simulink model "FaultCheck"  (R2022b)
settings: Solver=FixedStepAuto  StartTime=0.0  StopTime=10  FixedStep=1  RelTol=1e-3
undefined symbols (not defined in the file): C_Flt_IGBTULowerTempConfirmTh_u16, C_Flt_IGBTULowerTempDiagEn_b, C_Flt_IGBTULowerTempErrCode_u16, C_Flt_IGBTULowerTempPowerCoeff, C_Flt_IGBTULowerTempRecoveryTh_u16, C_Flt_IGBTULowerTempRecTh_s32, C_Flt_IGBTULowerTempTrigTh_s32, C_Flt_IGBTUOverTempConfirmTh_u16, C_Flt_IGBTUOverTempDiagEn_b, C_Flt_IGBTUOverTempErrCode_u16, C_Flt_IGBTUOverTempRecoveryTh_u16, C_Flt_IGBTUOverTempRecTh_s32, C_Flt_IGBTUOverTempTrigTh_s32, C_Flt_IGBTVLowerTempConfirmTh_u16, C_Flt_IGBTVLowerTempDiagEn_b, C_Flt_IGBTVLowerTempErrCode_u16, C_Flt_IGBTVLowerTempPowerCoeff, C_Flt_IGBTVLowerTempRecoveryTh_u16, C_Flt_IGBTVLowerTempRecTh_s32, C_Flt_IGBTVLowerTempTrigTh_s32, C_Flt_IGBTVOverTempConfirmTh_u16, C_Flt_IGBTVOverTempDiagEn_b, C_Flt_IGBTVOverTempErrCode_u16, C_Flt_IGBTVOverTempRecoveryTh_u16, C_Flt_IGBTVOverTempRecTh_s32, C_Flt_IGBTVOverTempTrigTh_s32, C_Flt_IGBTWLowerTempConfirmTh_u16, C_Flt_IGBTWLowerTempDiagEn_b, C_Flt_IGBTWLowerTempErrCode_u16, C_Flt_IGBTWLowerTempPowerCoeff, C_Flt_IGBTWLowerTempRecoveryTh_u16, C_Flt_IGBTWLowerTempRecTh_s32, C_Flt_IGBTWLowerTempTrigTh_s32, C_Flt_IGBTWOverTempConfirmTh_u16, C_Flt_IGBTWOverTempDiagEn_b, C_Flt_IGBTWOverTempErrCode_u16, C_Flt_IGBTWOverTempRecoveryTh_u16, C_Flt_IGBTWOverTempRecTh_s32, C_Flt_IGBTWOverTempTrigTh_s32, C_Flt_IuOCConfirmTh_u16, C_Flt_IuOCDiagEn_b, C_Flt_IuOCErrCode_u16, C_Flt_IuOCNegLimit_s32, C_Flt_IuOCPosLimit_s32, C_Flt_IuOCRecoveryTh_u16, C_Flt_IuZeroDriftDiagEn_b, C_Flt_IuZeroDriftErrCode_u16, C_Flt_IvOCConfirmTh_u16, C_Flt_IvOCDiagEn_b, C_Flt_IvOCErrCode_u16, C_Flt_IvOCNegLimit_s32, C_Flt_IvOCPosLimit_s32, C_Flt_IvOCRecoveryTh_u16, C_Flt_IvZeroDriftDiagEn_b, C_Flt_IvZeroDriftErrCode_u16, C_Flt_IwOCConfirmTh_u16, C_Flt_IwOCDiagEn_b, C_Flt_IwOCErrCode_u16, C_Flt_IwOCNegLimit_s32, C_Flt_IwOCPosLimit_s32 ... (+196)
libraries: YS_UserDefined_Library x21, simulink x5
(part 4 of 11)

== system FaultCheck/FaultDiag_HighTask_100us/FltDetn/UdcDetn/Parameter2 ==
  IPC_UdcRaw_V : Inport
  Bus Creator : BusCreator  Inputs=8
  Constant11 : Constant  Value=Flt_UdcOverLim1_ErrCode
  Constant13 : Constant  Value=FLTLVL_TWO
  Constant2 : Constant  Value=Flt_UdcOverLim1_RecLim1
  Constant3 : Constant  Value=Flt_UdcOverLim1_RecDeb
  Constant6 : Constant  Value=Flt_UdcOverLim1_ActvErrDetn
  Constant7 : Constant  Value=Flt_UdcOverLim1_OverLim1
  Constant8 : Constant  Value=Flt_UdcOverLim1_ErrDeb
  Flt_UdcOverLim1_PowRecCoef : Lookup_n-D  NumberOfTableDimensions=1  BreakpointsForDimension1=Flt_UdcRawOver1_V  BreakpointsForDimension1DataTypeStr=Inherit: Inherit from 'Breakpoint data'  Table=Flt_UdcOverLim1_PowRecCoef  TableDataTypeStr=Inherit: Inherit from 'Table data'  ExtrapMethod=Clip  UseLastTableValue=on  InternalRulePriority=Speed  OutDataTypeStr=single  RndMeth=Simplest
  Para : Outport
  wires:
  IPC_UdcRaw_V/1 -> Flt_UdcOverLim1_PowRecCoef/1
  Bus Creator/1 -> Para/1
  Constant11/1 -> Bus Creator/6  "ErrCode"
  Constant13/1 -> Bus Creator/7  "FltLvl"
  Flt_UdcOverLim1_PowRecCoef/1 -> Bus Creator/8  "PowRecCoef"
  Constant7/1 -> Bus Creator/1  "OverLim1"
  Constant8/1 -> Bus Creator/2  "ErrDeb"
  Constant6/1 -> Bus Creator/3  "ActvnDetn"
  Constant3/1 -> Bus Creator/5  "RecDeb"
  Constant2/1 -> Bus Creator/4  "RecLim1"

== system FaultCheck/FaultDiag_HighTask_100us/FltDetn/UdcDetn/Parameter3 ==
  Bus Creator : BusCreator  Inputs=6
  Constant1 : Constant  Value=FLT_COEF_ZERO
  Constant11 : Constant  Value=Flt_UdcOverLim2_ErrCode
  Constant13 : Constant  Value=FLTLVL_FIVE
  Constant6 : Constant  Value=Flt_UdcOverLim2_ActvErrDetn
  Constant7 : Constant  Value=Flt_UdcOverLim2_OverLim2
  Constant8 : Constant  Value=Flt_UdcOverLim2_ErrDeb
  Para : Outport
  wires:
  Bus Creator/1 -> Para/1
  Constant11/1 -> Bus Creator/4  "ErrCode"
  Constant13/1 -> Bus Creator/5  "FltLvl"
  Constant1/1 -> Bus Creator/6  "PowRecCoef"
  Constant7/1 -> Bus Creator/1  "OverLim2"
  Constant8/1 -> Bus Creator/2  "ErrDeb"
  Constant6/1 -> Bus Creator/3  "ActvnDetn"

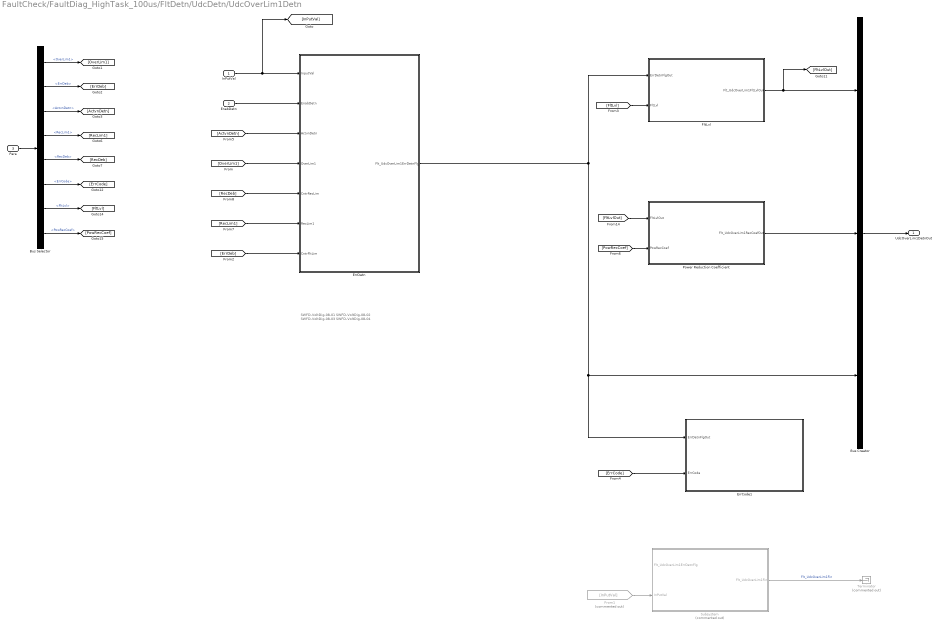
== system FaultCheck/FaultDiag_HighTask_100us/FltDetn/UdcDetn/UdcOverLim1Detn ==
  note: SWFD-VoltDig-08-01
      |
      | SWFD-VoltDig-08-02
      |
      | SWFD-VoltDig-08-03
      |
      | SWFD-VoltDig-08-04
  InPutVal : Inport
  EnabDetn : Inport  Port=2
  Para : Inport  Port=3
  Bus Creator : BusCreator  Inputs=3
  Bus Selector : BusSelector  OutputSignals=OverLim1,ErrDeb,ActvnDetn,RecLim1,RecDeb,ErrCode,FltLvl,PowRecCoef
  ErrCode1 : Subsystem
  ErrDetn : Subsystem
  FltLvl : Subsystem
  From1 : From  Commented=on  GotoTag=InPutVal
  Power Reduction Coefficient : Subsystem
  Subsystem : Subsystem  Commented=on
  Terminator : Terminator  Commented=on
  UdcOverLim1DetnOut : Outport
  wires:
  ErrDetn/1(Flt_UdcOverLim1ErrDetnFlg) -> FltLvl/1(ErrDetnFlgOut), Bus Creator/3, ErrCode1/1(ErrDetnFlgOut)
  Subsystem/1(Flt_UdcOverLim1Fin) -> Terminator/1  "Flt_UdcOverLim1Fin"
  From1/1 -> Subsystem/2(InPutVal)
  Bus Selector/1 -> [OverLim1]  "<OverLim1>"
  Para/1 -> Bus Selector/1
  Bus Selector/3 -> [ActvnDetn]  "<ActvnDetn>"
  Bus Selector/2 -> [ErrDeb]  "<ErrDeb>"
  Bus Selector/4 -> [RecLim1]  "<RecLim1>"
  Bus Selector/5 -> [RecDeb]  "<RecDeb>"
  FltLvl/1(Flt_UdcOverLim1FltLvlOut) -> Bus Creator/1, [FltLvlOut]
  Bus Selector/6 -> [ErrCode]  "<ErrCode>"
  Bus Selector/7 -> [FltLvl]  "<FltLvl>"
  Bus Selector/8 -> [PowRecCoef]  "<PowRecCoef>"
  [FltLvl] -> FltLvl/2(FltLvl)
  [PowRecCoef] -> Power Reduction Coefficient/2(PowRecCoef)
  [FltLvlOut] -> Power Reduction Coefficient/1(FltLvlOut)
  InPutVal/1 -> ErrDetn/1(InputVal), [InPutVal]
  [OverLim1] -> ErrDetn/4(OverLim1)
  EnabDetn/1 -> ErrDetn/2(EnabDetn)
  [ActvnDetn] -> ErrDetn/3(ActvnDetn)
  Power Reduction Coefficient/1(Flt_UdcOverLim1RecCoefOut) -> Bus Creator/2
  Bus Creator/1 -> UdcOverLim1DetnOut/1
  [RecDeb] -> ErrDetn/5(CntrRecLim)
  [RecLim1] -> ErrDetn/6(RecLim1)
  [ErrDeb] -> ErrDetn/7(CntrFltLim)
  [ErrCode] -> ErrCode1/2(ErrCode)

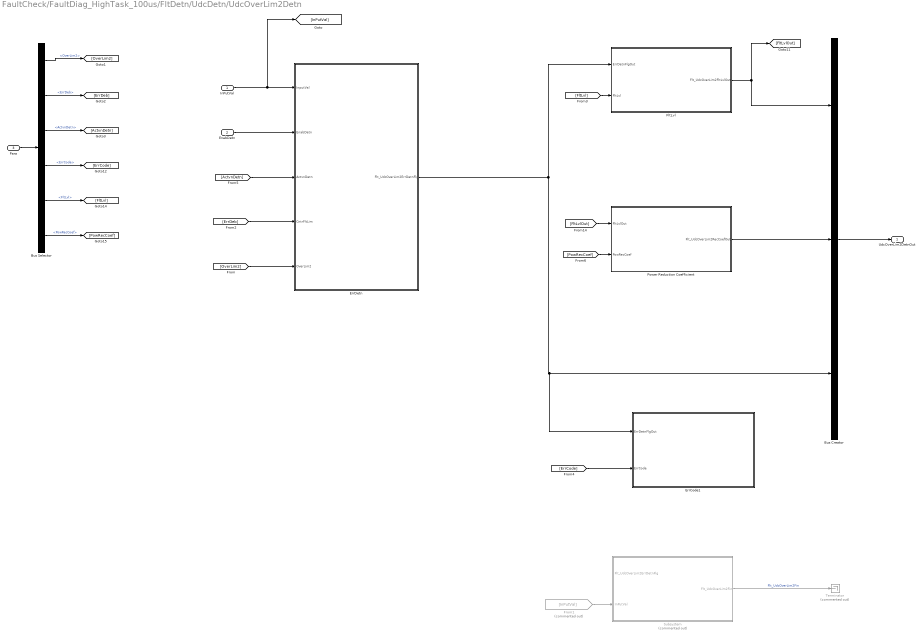
== system FaultCheck/FaultDiag_HighTask_100us/FltDetn/UdcDetn/UdcOverLim2Detn ==
  InPutVal : Inport
  EnabDetn : Inport  Port=2
  Para : Inport  Port=3
  Bus Creator : BusCreator  Inputs=3
  Bus Selector : BusSelector  OutputSignals=OverLim2,ErrDeb,ActvnDetn,ErrCode,FltLvl,PowRecCoef
  ErrCode1 : Subsystem
  ErrDetn : Subsystem
  FltLvl : Subsystem
  From1 : From  Commented=on  GotoTag=InPutVal
  Power Reduction Coefficient : Subsystem
  Subsystem : Subsystem  Commented=on
  Terminator : Terminator  Commented=on
  UdcOverLim2DetnOut : Outport
  wires:
  ErrDetn/1(Flt_UdcOverLim2ErrDetnFlg) -> ErrCode1/1(ErrDetnFlgOut), Bus Creator/3, FltLvl/1(ErrDetnFlgOut)
  From1/1 -> Subsystem/2(InPutVal)
  Subsystem/1(Flt_UdcOverLim2Fin) -> Terminator/1  "Flt_UdcOverLim2Fin"
  [ErrDeb] -> ErrDetn/4(CntrFltLim)
  Bus Creator/1 -> UdcOverLim2DetnOut/1
  Power Reduction Coefficient/1(Flt_UdcOverLim2RecCoefOut) -> Bus Creator/2
  [ActvnDetn] -> ErrDetn/3(ActvnDetn)
  EnabDetn/1 -> ErrDetn/2(EnabDetn)
  [OverLim2] -> ErrDetn/5(OverLim2)
  InPutVal/1 -> ErrDetn/1(InputVal), [InPutVal]
  [FltLvlOut] -> Power Reduction Coefficient/1(FltLvlOut)
  [PowRecCoef] -> Power Reduction Coefficient/2(PowRecCoef)
  [FltLvl] -> FltLvl/2(FltLvl)
  Bus Selector/6 -> [PowRecCoef]  "<PowRecCoef>"
  Bus Selector/5 -> [FltLvl]  "<FltLvl>"
  Bus Selector/4 -> [ErrCode]  "<ErrCode>"
  FltLvl/1(Flt_UdcOverLim2FltLvlOut) -> [FltLvlOut], Bus Creator/1
  Bus Selector/2 -> [ErrDeb]  "<ErrDeb>"
  Bus Selector/3 -> [ActvnDetn]  "<ActvnDetn>"
  Bus Selector/1 -> [OverLim2]  "<OverLim2>"
  Para/1 -> Bus Selector/1
  [ErrCode] -> ErrCode1/2(ErrCode)

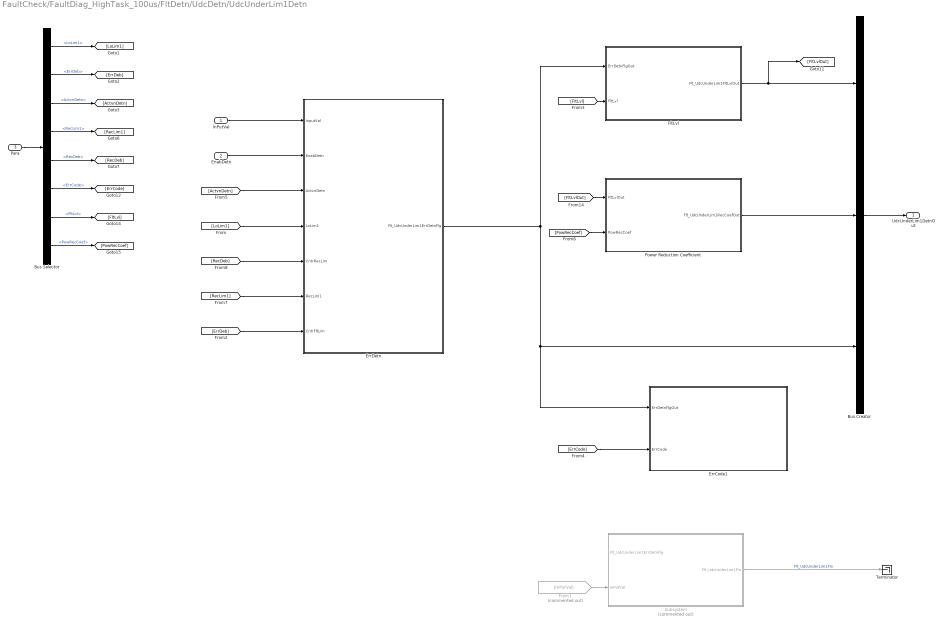
== system FaultCheck/FaultDiag_HighTask_100us/FltDetn/UdcDetn/UdcUnderLim1Detn ==
  InPutVal : Inport
  EnabDetn : Inport  Port=2
  Para : Inport  Port=3
  Bus Creator : BusCreator  Inputs=3
  Bus Selector : BusSelector  OutputSignals=LoLim1,ErrDeb,ActvnDetn,RecLim1,RecDeb,ErrCode,FltLvl,PowRecCoef
  ErrCode1 : Subsystem
  ErrDetn : Subsystem
  FltLvl : Subsystem
  From1 : From  Commented=on  GotoTag=InPutVal
  Power Reduction Coefficient : Subsystem
  Subsystem : Subsystem  Commented=on
  Terminator : Terminator
  UdcUnderLim1DetnOut : Outport
  wires:
  Subsystem/1(Flt_UdcUnderLim1Fin) -> Terminator/1  "Flt_UdcUnderLim1Fin"
  From1/1 -> Subsystem/2(InPutVal)
  ErrDetn/1(Flt_UdcUnderLim1ErrDetnFlg) -> Bus Creator/3, ErrCode1/1(ErrDetnFlgOut), FltLvl/1(ErrDetnFlgOut)
  [ErrDeb] -> ErrDetn/7(CntrFltLim)
  [RecLim1] -> ErrDetn/6(RecLim1)
  [RecDeb] -> ErrDetn/5(CntrRecLim)
  Bus Creator/1 -> UdcUnderLim1DetnOut/1
  Power Reduction Coefficient/1(Flt_UdcUnderLim1RecCoefOut) -> Bus Creator/2
  [ActvnDetn] -> ErrDetn/3(ActvnDetn)
  EnabDetn/1 -> ErrDetn/2(EnabDetn)
  [LoLim1] -> ErrDetn/4(LoLim1)
  InPutVal/1 -> ErrDetn/1(InputVal)
  [FltLvlOut] -> Power Reduction Coefficient/1(FltLvlOut)
  [PowRecCoef] -> Power Reduction Coefficient/2(PowRecCoef)
  [FltLvl] -> FltLvl/2(FltLvl)
  Bus Selector/8 -> [PowRecCoef]  "<PowRecCoef>"
  Bus Selector/7 -> [FltLvl]  "<FltLvl>"
  Bus Selector/6 -> [ErrCode]  "<ErrCode>"
  FltLvl/1(Flt_UdcUnderLim1FltLvlOut) -> Bus Creator/1, [FltLvlOut]
  Bus Selector/5 -> [RecDeb]  "<RecDeb>"
  Bus Selector/4 -> [RecLim1]  "<RecLim1>"
  Bus Selector/2 -> [ErrDeb]  "<ErrDeb>"
  Bus Selector/3 -> [ActvnDetn]  "<ActvnDetn>"
  Bus Selector/1 -> [LoLim1]  "<LoLim1>"
  Para/1 -> Bus Selector/1
  [ErrCode] -> ErrCode1/2(ErrCode)

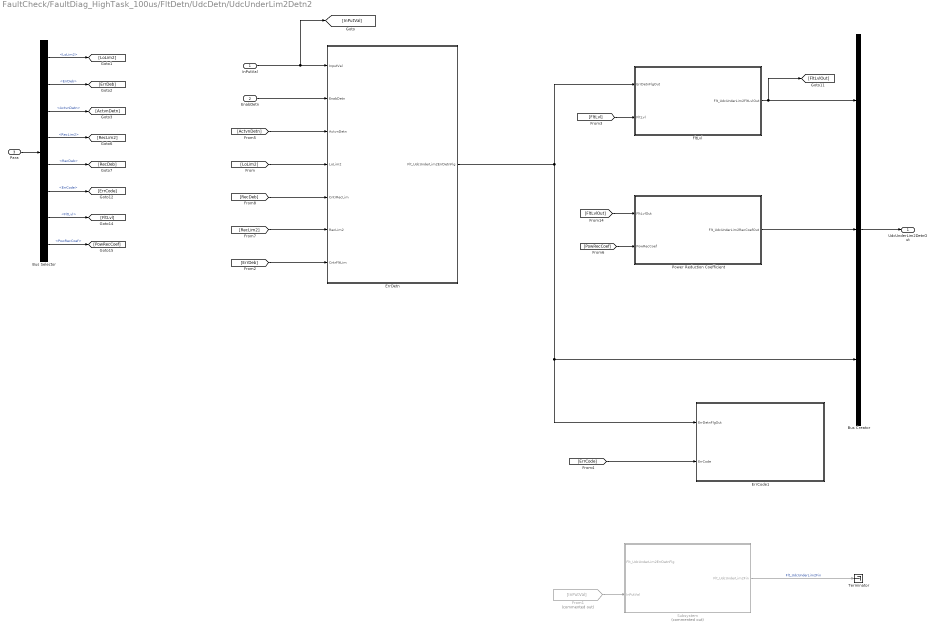
== system FaultCheck/FaultDiag_HighTask_100us/FltDetn/UdcDetn/UdcUnderLim2Detn2 ==
  InPutVal : Inport
  EnabDetn : Inport  Port=2
  Para : Inport  Port=3
  Bus Creator : BusCreator  Inputs=3
  Bus Selector : BusSelector  OutputSignals=LoLim2,ErrDeb,ActvnDetn,RecLim2,RecDeb,ErrCode,FltLvl,PowRecCoef
  ErrCode1 : Subsystem
  ErrDetn : Subsystem
  FltLvl : Subsystem
  From1 : From  Commented=on  GotoTag=InPutVal
  Power Reduction Coefficient : Subsystem
  Subsystem : Subsystem  Commented=on
  Terminator : Terminator
  UdcUnderLim2DetnOut : Outport
  wires:
  From1/1 -> Subsystem/2(InPutVal)
  Subsystem/1(Flt_UdcUnderLim2Fin) -> Terminator/1  "Flt_UdcUnderLim2Fin"
  Para/1 -> Bus Selector/1
  Bus Selector/1 -> [LoLim2]  "<LoLim2>"
  Bus Selector/3 -> [ActvnDetn]  "<ActvnDetn>"
  Bus Selector/2 -> [ErrDeb]  "<ErrDeb>"
  Bus Selector/4 -> [RecLim2]  "<RecLim2>"
  Bus Selector/5 -> [RecDeb]  "<RecDeb>"
  ErrDetn/1(Flt_UdcUnderLim2ErrDetnFlg) -> FltLvl/1(ErrDetnFlgOut), Bus Creator/3, ErrCode1/1(ErrDetnFlgOut)
  FltLvl/1(Flt_UdcUnderLim2FltLvlOut) -> Bus Creator/1, [FltLvlOut]
  Bus Selector/6 -> [ErrCode]  "<ErrCode>"
  Bus Selector/7 -> [FltLvl]  "<FltLvl>"
  Bus Selector/8 -> [PowRecCoef]  "<PowRecCoef>"
  [FltLvl] -> FltLvl/2(FltLvl)
  [PowRecCoef] -> Power Reduction Coefficient/2(PowRecCoef)
  [FltLvlOut] -> Power Reduction Coefficient/1(FltLvlOut)
  InPutVal/1 -> ErrDetn/1(InputVal), [InPutVal]
  [LoLim2] -> ErrDetn/4(LoLim2)
  EnabDetn/1 -> ErrDetn/2(EnabDetn)
  [ActvnDetn] -> ErrDetn/3(ActvnDetn)
  Power Reduction Coefficient/1(Flt_UdcUnderLim2RecCoefOut) -> Bus Creator/2
  Bus Creator/1 -> UdcUnderLim2DetnOut/1
  [RecDeb] -> ErrDetn/5(CntrRecLim)
  [RecLim2] -> ErrDetn/6(RecLim2)
  [ErrDeb] -> ErrDetn/7(CntrFltLim)
  [ErrCode] -> ErrCode1/2(ErrCode)

== system FaultCheck/FaultDiag_HighTask_100us/FltDetn/UdcZeroDrfDetn/Enable ==
  Constant : Constant  Value=FLT_ON
  Enable : Outport
  wires:
  Constant/1 -> Enable/1

== system FaultCheck/FaultDiag_HighTask_100us/FltDetn/UdcZeroDrfDetn/Parameter ==
  Bus Creator : BusCreator  Inputs=4
  Constant2 : Constant  Value=FLT_COEF_ZERO
  Constant3 : Constant  Value=Flt_UdcZeroDrf_ErrCode
  Constant4 : Constant  Value=FLTLVL_FIVE
  Constant5 : Constant  Value=Flt_UdcZeroDrf_ActvnErrDetn
  Para : Outport
  wires:
  Constant2/1 -> Bus Creator/4  "PowRecCoef"
  Constant3/1 -> Bus Creator/2  "ErrCode"
  Constant5/1 -> Bus Creator/1  "ActvnDetn"
  Constant4/1 -> Bus Creator/3  "FltLvl"
  Bus Creator/1 -> Para/1

== system FaultCheck/FaultDiag_HighTask_100us/FltDetn/UdcZeroDrfDetn/UdcZeroDrfDetn ==
  InPutVal : Inport
  EnabDetn : Inport  Port=2
  Para : Inport  Port=3
  Bus Selector : BusSelector  OutputSignals=ActvnDetn,ErrCode,FltLvl,PowRecCoef
  ErrCode1 : Subsystem
  ErrDetn : Subsystem
  FltLvl : Subsystem
  Power Reduction Coefficient : Subsystem
  Flt_UdcZeroDrfFltLvl : Outport
  Flt_UdcZeroDrfPowRecCoefOut : Outport  Port=2
  wires:
  ErrDetn/1(Flt_UdcZeroDrfErrFlg) -> FltLvl/1(ErrDetnFlgOut), ErrCode1/1(ErrDetnFlgOut)
  InPutVal/1 -> ErrDetn/1(InputVal)
  [ActvnDetn] -> ErrDetn/3(ActvnDetn)
  EnabDetn/1 -> ErrDetn/2(EnabDetn)
  Bus Selector/4 -> [PowRecCoef]  "<PowRecCoef>"
  Bus Selector/3 -> [FltLvl]  "<FltLvl>"
  Bus Selector/2 -> [ErrCode]  "<ErrCode>"
  Bus Selector/1 -> [ActvnDetn]  "<ActvnDetn>"
  Para/1 -> Bus Selector/1
  [ErrCode] -> ErrCode1/2(ErrCode)
  FltLvl/1(Flt_UdcZeroDrfFltLvl) -> [FltLvlOut], Flt_UdcZeroDrfFltLvl/1
  [FltLvl] -> FltLvl/2(FltLvl)
  [FltLvlOut] -> Power Reduction Coefficient/1(FltLvlOut)
  [PowRecCoef] -> Power Reduction Coefficient/2(PowRecCoef)
  Power Reduction Coefficient/1(Flt_UdcZeroDrfPowRecCoefOut) -> Flt_UdcZeroDrfPowRecCoefOut/1

== system FaultCheck/FaultDiag_HighTask_100us/FltDetn/VoltagSensorDetn/Enable ==
  Sys_SelfChkFishFlg : Inport
  Constant : Constant  Value=FLT_ON
  Constant1 : Constant  Value=FLT_ON
  Constant2 : Constant  Value=FLT_OFF
  Relational Operator : RelationalOperator  Operator===  OutDataTypeStr=boolean  RndMeth=Simplest  InputSameDT=off
  Switch : Switch  Criteria=u2 > Threshold  SaturateOnIntegerOverflow=off  InputSameDT=off
  Enable : Outport
  wires:
  Switch/1 -> Enable/1
  Constant2/1 -> Switch/3
  Constant1/1 -> Switch/1
  Relational Operator/1 -> Switch/2
  Constant/1 -> Relational Operator/2
  Sys_SelfChkFishFlg/1 -> Relational Operator/1

== system FaultCheck/FaultDiag_HighTask_100us/FltDetn/VoltagSensorDetn/Flt_VoltagSensorDetn ==
  InPutVal1 : Inport
  EnabDetn : Inport  Port=2
  Para : Inport  Port=3
  IPT_UdcRaw_mV : Inport  Port=4
  Bus Selector : BusSelector  OutputSignals=ActvnDetn,ErrCode,FltLvl,PowRecCoef,ErrDeb
  Data Type Conversion : DataTypeConversion  OutDataTypeStr=fixdt('uint16', 'DataTypeOverride', 'Off')  SaturateOnIntegerOverflow=off  RndMeth=Floor
  ErrCode : Subsystem
  ErrDetn : Subsystem
  FltLvl : Subsystem
  Power Reduction Coefficient : Subsystem
  Subsystem : Subsystem
  Terminator : Terminator
  Flt_VoltagSensorFltLvl : Outport
  Flt_VoltagSensorPowRecCoefOut : Outport  Port=2
  wires:
  IPT_UdcRaw_mV/1 -> Subsystem/2(IPT_UdcRaw_mV)
  Subsystem/1(Flt_VoltagSensorFin) -> Terminator/1  "Flt_VoltagSensorFin"
  ErrDetn/1(FFlt_VoltagSensorErrFlg) -> Subsystem/1(Flt_VoltagSensorErrDetnFlg), FltLvl/1(ErrDetnFlgOut), ErrCode/1(ErrDetnFlgOut)
  Bus Selector/5 -> [ErrDeb]  "<ErrDeb>"
  InPutVal1/1 -> ErrDetn/1(InputVal)
  [ActvnDetn] -> ErrDetn/3(ActvnDetn)
  EnabDetn/1 -> ErrDetn/2(EnabDetn)
  [ErrDeb] -> ErrDetn/4(ErrDeb)
  Bus Selector/4 -> [PowRecCoef]  "<PowRecCoef>"
  Bus Selector/3 -> [FltLvl]  "<FltLvl>"
  Bus Selector/2 -> [ErrCode]  "<ErrCode>"
  Bus Selector/1 -> [ActvnDetn]  "<ActvnDetn>"
  Para/1 -> Bus Selector/1
  [ErrCode] -> Data Type Conversion/1
  FltLvl/1(Flt_VoltagSensorFltLvl) -> [FltLvlOut], Flt_VoltagSensorFltLvl/1
  [FltLvl] -> FltLvl/2(FltLvl)
  [FltLvlOut] -> Power Reduction Coefficient/1(FltLvlOut)
  [PowRecCoef] -> Power Reduction Coefficient/2(PowRecCoef)
  Power Reduction Coefficient/1(Flt_VoltagSensorPowRecCoefOut) -> Flt_VoltagSensorPowRecCoefOut/1
  Data Type Conversion/1 -> ErrCode/2(ErrCode)

== system FaultCheck/FaultDiag_HighTask_100us/FltDetn/VoltagSensorDetn/Parameter ==
  Bus Creator : BusCreator  Inputs=5
  Constant2 : Constant  Value=FLT_COEF_ZERO
  Constant3 : Constant  Value=Flt_VoltagSensor_ErrCode
  Constant4 : Constant  Value=FLTLVL_FOUR
  Constant5 : Constant  Value=Flt_VoltagSensor_ActvnDetn
  Constant8 : Constant  Value=Flt_VoltagSensor_ErrDeb
  Para : Outport
  wires:
  Constant8/1 -> Bus Creator/1  "ErrDeb"
  Constant2/1 -> Bus Creator/5  "PowRecCoef"
  Constant3/1 -> Bus Creator/3  "ErrCode"
  Constant5/1 -> Bus Creator/2  "ActvnDetn"
  Constant4/1 -> Bus Creator/4  "FltLvl"
  Bus Creator/1 -> Para/1

== system FaultCheck/FaultDiag_HighTask_100us/FltHandle/ValOut/CurrentVal ==
  FltSignalBus : Inport
  Bus Selector : BusSelector  OutputSignals=IPC_IuRaw_A,IPC_IvRaw_A,IPC_IwRaw_A
  Flt_IuOut_A : Outport
  Flt_IvOut_A : Outport  Port=2
  Flt_IwOut_A1 : Outport  Port=3
  wires:
  FltSignalBus/1 -> Bus Selector/1
  Bus Selector/1 -> Flt_IuOut_A/1  "<IPC_IuRaw_A>"
  Bus Selector/2 -> Flt_IvOut_A/1  "<IPC_IvRaw_A>"
  Bus Selector/3 -> Flt_IwOut_A1/1  "<IPC_IwRaw_A>"

== system FaultCheck/FaultDiagnose/CurrZeroDriftFltDiag/IuZeroDriftDiag/Diagnose ==
  IuZeroDftEn : Inport
  IuZeroDriftFltFlg : Inport  Port=2
  SysSelfCheckDownFlg : Inport  Port=3
  Disable : Subsystem  TreatAsAtomicUnit=on
  If : If  IfExpression=u1 == 0
  Merge : Merge
  Normal : Subsystem  TreatAsAtomicUnit=on
  Subsystem : Subsystem
  IuZeroDriftFltFlgOut : Outport
  wires:
  If/1 -> Disable/Action
  If/2 -> Normal/Action
  Disable/1(FlgOut) -> Merge/1
  Normal/1(FlgOut) -> Merge/2
  IuZeroDriftFltFlg/1 -> Normal/1(IuZeroDriftFltFlg)
  Merge/1 -> IuZeroDriftFltFlgOut/1  "M_Flt_IuZeroDriftFltFlgOut_b"
  IuZeroDftEn/1 -> Subsystem/1(IuZeroDftEn)
  SysSelfCheckDownFlg/1 -> Subsystem/2(SysSelfCheckDownFlg)
  Subsystem/1(IuZeroDriftDiagEn) -> If/1

== system FaultCheck/FaultDiagnose/CurrZeroDriftFltDiag/IuZeroDriftDiag/FaultLevelDeter ==
  IuZeroDriftFltFlgOut : Inport
  FaultLevel : Inport  Port=2
  If : If  IfExpression=u1 == 0
  Merge : Merge
  Normal : Subsystem  TreatAsAtomicUnit=on
  ZeroDriftFlt : Subsystem  TreatAsAtomicUnit=on
  IuZeroDriftFltLevelOut : Outport
  wires:
  IuZeroDriftFltFlgOut/1 -> If/1
  If/1 -> Normal/Action
  If/2 -> ZeroDriftFlt/Action
  FaultLevel/1 -> ZeroDriftFlt/1(FaultLevel)
  Normal/1(IuZeroDriftFltLevel) -> Merge/1
  ZeroDriftFlt/1(IuZeroDriftFltLevel) -> Merge/2
  Merge/1 -> IuZeroDriftFltLevelOut/1  "M_Flt_IuZeroDriftFltLevelOut_u8"

== system FaultCheck/FaultDiagnose/CurrZeroDriftFltDiag/IuZeroDriftDiag/Parameters ==
  Bus Creator : BusCreator  Inputs=4
  Constant : Constant  Value=C_Flt_IuZeroDriftDiagEn_b
  Constant1 : Constant  Value=C_Flt_IuZeroDriftErrCode_u16
  Constant2 : Constant  Value=C_Flt_LevelFive_u8
  Constant3 : Constant  Value=C_Flt_PowerCoeffZero_s32
  IuZeroDriftParam : Outport
  wires:
  Constant/1 -> Bus Creator/1  "IuZeroDriftDiagEn"
  Constant1/1 -> Bus Creator/2  "IuZeroDriftErrCode"
  Constant2/1 -> Bus Creator/3  "IuZeroDriftFltLevel"
  Constant3/1 -> Bus Creator/4  "IuZeroDriftPowerCoeff"
  Bus Creator/1 -> IuZeroDriftParam/1

== system FaultCheck/FaultDiagnose/CurrZeroDriftFltDiag/IuZeroDriftDiag/PowerReductionCoeffDeter ==
  IuZeroDriftFltLevelOut : Inport
  PowerCoeff : Inport  Port=2
  If : If  IfExpression=u1 < 2  ElseIfExpressions=u1 == 2
  If Action Subsystem : Subsystem  TreatAsAtomicUnit=on
  If Action Subsystem1 : Subsystem  TreatAsAtomicUnit=on
  If Action Subsystem2 : Subsystem  TreatAsAtomicUnit=on
  Merge : Merge  Inputs=3
  IuZeroDriftPowerCoeff : Outport
  wires:
  IuZeroDriftFltLevelOut/1 -> If/1
  If/1 -> If Action Subsystem/Action
  If/2 -> If Action Subsystem1/Action
  If/3 -> If Action Subsystem2/Action
  PowerCoeff/1 -> If Action Subsystem1/1(PowerCoeff)
  If Action Subsystem/1(Coeff) -> Merge/1
  If Action Subsystem1/1(Coeff) -> Merge/2
  If Action Subsystem2/1(Coeff) -> Merge/3
  Merge/1 -> IuZeroDriftPowerCoeff/1  "M_Flt_IuZeroDriftPowerCoeffOut_s32"

== system FaultCheck/FaultDiagnose/CurrZeroDriftFltDiag/IvZeroDriftDiag/Diagnose ==
  IvZeroDftEn : Inport
  IvZeroDriftFltFlg : Inport  Port=2
  SysSelfCheckDownFlg : Inport  Port=3
  Disable : Subsystem  TreatAsAtomicUnit=on
  If : If  IfExpression=u1 == 0
  Merge : Merge
  Normal : Subsystem  TreatAsAtomicUnit=on
  Subsystem : Subsystem
  IvZeroDriftFltFlgOut : Outport
  wires:
  Merge/1 -> IvZeroDriftFltFlgOut/1  "M_Flt_IvZeroDriftFltFlgOut_b"
  IvZeroDriftFltFlg/1 -> Normal/1(IvZeroDriftFltFlg)
  Normal/1(FlgOut) -> Merge/2
  Disable/1(FlgOut) -> Merge/1
  If/2 -> Normal/Action
  If/1 -> Disable/Action
  IvZeroDftEn/1 -> Subsystem/1(IvZeroDftEn)
  SysSelfCheckDownFlg/1 -> Subsystem/2(SysSelfCheckDownFlg)
  Subsystem/1(IvZeroDriftDiagEn) -> If/1

== system FaultCheck/FaultDiagnose/CurrZeroDriftFltDiag/IvZeroDriftDiag/FaultLevelDeter ==
  IvZeroDriftFltFlgOut : Inport
  FaultLevel : Inport  Port=2
  If : If  IfExpression=u1 == 0
  Merge : Merge
  Normal : Subsystem  TreatAsAtomicUnit=on
  ZeroDriftFlt : Subsystem  TreatAsAtomicUnit=on
  IvZeroDriftFltLevelOut : Outport
  wires:
  Merge/1 -> IvZeroDriftFltLevelOut/1  "M_Flt_IvZeroDriftFltLevelOut_u8"
  ZeroDriftFlt/1(IvZeroDriftFltLevel) -> Merge/2
  Normal/1(IvZeroDriftFltLevel) -> Merge/1
  FaultLevel/1 -> ZeroDriftFlt/1(FaultLevel)
  If/2 -> ZeroDriftFlt/Action
  If/1 -> Normal/Action
  IvZeroDriftFltFlgOut/1 -> If/1

== system FaultCheck/FaultDiagnose/CurrZeroDriftFltDiag/IvZeroDriftDiag/Parameters ==
  Bus Creator : BusCreator  Inputs=4
  Constant : Constant  Value=C_Flt_IvZeroDriftDiagEn_b
  Constant1 : Constant  Value=C_Flt_IvZeroDriftErrCode_u16
  Constant2 : Constant  Value=C_Flt_LevelFive_u8
  Constant3 : Constant  Value=C_Flt_PowerCoeffZero_s32
  IvZeroDriftParam : Outport
  wires:
  Bus Creator/1 -> IvZeroDriftParam/1
  Constant3/1 -> Bus Creator/4  "IvZeroDriftPowerCoeff"
  Constant2/1 -> Bus Creator/3  "IvZeroDriftFltLevel"
  Constant1/1 -> Bus Creator/2  "IvZeroDriftErrCode"
  Constant/1 -> Bus Creator/1  "IvZeroDriftDiagEn"

== system FaultCheck/FaultDiagnose/CurrZeroDriftFltDiag/IvZeroDriftDiag/PowerReductionCoeffDeter ==
  IvZeroDriftFltLevelOut : Inport
  PowerCoeff : Inport  Port=2
  If : If  IfExpression=u1 < 2  ElseIfExpressions=u1 == 2
  If Action Subsystem : Subsystem  TreatAsAtomicUnit=on
  If Action Subsystem1 : Subsystem  TreatAsAtomicUnit=on
  If Action Subsystem2 : Subsystem  TreatAsAtomicUnit=on
  Merge : Merge  Inputs=3
  IvZeroDriftPowerCoeff : Outport
  wires:
  Merge/1 -> IvZeroDriftPowerCoeff/1  "M_Flt_IvZeroDriftPowerCoeffOut_s32"
  If Action Subsystem2/1(Coeff) -> Merge/3
  If Action Subsystem1/1(Coeff) -> Merge/2
  If Action Subsystem/1(Coeff) -> Merge/1
  PowerCoeff/1 -> If Action Subsystem1/1(PowerCoeff)
  If/3 -> If Action Subsystem2/Action
  If/2 -> If Action Subsystem1/Action
  If/1 -> If Action Subsystem/Action
  IvZeroDriftFltLevelOut/1 -> If/1

== system FaultCheck/FaultDiagnose/CurrZeroDriftFltDiag/IwZeroDriftDiag/Diagnose ==
  IwZeroDftEn : Inport
  IwZeroDriftFltFlg : Inport  Port=2
  SysSelfCheckDownFlg : Inport  Port=3
  Disable : Subsystem  TreatAsAtomicUnit=on
  If : If  IfExpression=u1 == 0
  Merge : Merge
  Normal : Subsystem  TreatAsAtomicUnit=on
  Subsystem : Subsystem
  IwZeroDriftFltFlgOut : Outport
  wires:
  If/1 -> Disable/Action
  If/2 -> Normal/Action
  Disable/1(FlgOut) -> Merge/1
  Normal/1(FlgOut) -> Merge/2
  IwZeroDriftFltFlg/1 -> Normal/1(IwZeroDriftFltFlg)
  Merge/1 -> IwZeroDriftFltFlgOut/1  "M_Flt_IwZeroDriftFltFlgOut_b"
  SysSelfCheckDownFlg/1 -> Subsystem/2(SysSelfCheckDownFlg)
  IwZeroDftEn/1 -> Subsystem/1(IwZeroDftEn)
  Subsystem/1(IwZeroDriftDiagEn) -> If/1

== system FaultCheck/FaultDiagnose/CurrZeroDriftFltDiag/IwZeroDriftDiag/FaultLevelDeter ==
  IwZeroDriftFltFlgOut : Inport
  FaultLevel : Inport  Port=2
  If : If  IfExpression=u1 == 0
  Merge : Merge
  Normal : Subsystem  TreatAsAtomicUnit=on
  ZeroDriftFlt : Subsystem  TreatAsAtomicUnit=on
  IwZeroDriftFltLevelOut : Outport
  wires:
  IwZeroDriftFltFlgOut/1 -> If/1
  If/1 -> Normal/Action
  If/2 -> ZeroDriftFlt/Action
  FaultLevel/1 -> ZeroDriftFlt/1(FaultLevel)
  Normal/1(IwZeroDriftFltLevel) -> Merge/1
  ZeroDriftFlt/1(IwZeroDriftFltLevel) -> Merge/2
  Merge/1 -> IwZeroDriftFltLevelOut/1  "M_Flt_IwZeroDriftFltLevelOut_u8"

== system FaultCheck/FaultDiagnose/CurrZeroDriftFltDiag/IwZeroDriftDiag/Parameters ==
  Bus Creator : BusCreator  Inputs=4
  Constant : Constant  Value=C_Flt_IwZeroDriftDiagEn_b
  Constant1 : Constant  Value=C_Flt_IwZeroDriftErrCode_u16
  Constant2 : Constant  Value=C_Flt_LevelFive_u8
  Constant3 : Constant  Value=C_Flt_PowerCoeffZero_s32
  IwZeroDriftParam : Outport
  wires:
  Constant/1 -> Bus Creator/1  "IwZeroDriftDiagEn"
  Constant1/1 -> Bus Creator/2  "IwZeroDriftErrCode"
  Constant2/1 -> Bus Creator/3  "IwZeroDriftFltLevel"
  Constant3/1 -> Bus Creator/4  "IwZeroDriftPowerCoeff"
  Bus Creator/1 -> IwZeroDriftParam/1

== system FaultCheck/FaultDiagnose/CurrZeroDriftFltDiag/IwZeroDriftDiag/PowerReductionCoeffDeter ==
  IwZeroDriftFltLevelOut : Inport
  PowerCoeff : Inport  Port=2
  If : If  IfExpression=u1 < 2  ElseIfExpressions=u1 == 2
  If Action Subsystem : Subsystem  TreatAsAtomicUnit=on
  If Action Subsystem1 : Subsystem  TreatAsAtomicUnit=on
  If Action Subsystem2 : Subsystem  TreatAsAtomicUnit=on
  Merge : Merge  Inputs=3
  IwZeroDriftPowerCoeff : Outport
  wires:
  IwZeroDriftFltLevelOut/1 -> If/1
  If/1 -> If Action Subsystem/Action
  If/2 -> If Action Subsystem1/Action
  If/3 -> If Action Subsystem2/Action
  PowerCoeff/1 -> If Action Subsystem1/1(PowerCoeff)
  If Action Subsystem/1(Coeff) -> Merge/1
  If Action Subsystem1/1(Coeff) -> Merge/2
  If Action Subsystem2/1(Coeff) -> Merge/3
  Merge/1 -> IwZeroDriftPowerCoeff/1  "M_Flt_IwZeroDriftPowerCoeffOut_s32"

== system FaultCheck/FaultDiagnose/IGBTTempDiag/IGBTULowerTempDiag/Diagnose ==
  DiagEnOut : Inport
  IGBTUTemp : Inport  Port=2
  Parameter : Inport  Port=3
  Disable : Subsystem  TreatAsAtomicUnit=on
  If : If  IfExpression=u1 == 0
  Merge : Merge
  NormalDiag : Subsystem  TreatAsAtomicUnit=on
  IGBTULowerTempFlgOut : Outport
  wires:
  Merge/1 -> IGBTULowerTempFlgOut/1  "M_Flt_IGBTULowerTempFlgOut_b"
  NormalDiag/1(IGBTULowerTempFltDeb) -> Merge/2
  Disable/1(IGBTULowerTempFltDeb) -> Merge/1
  Parameter/1 -> NormalDiag/2(Parameter)
  IGBTUTemp/1 -> NormalDiag/1(IGBTUTemp)
  If/2 -> NormalDiag/Action
  If/1 -> Disable/Action
  DiagEnOut/1 -> If/1

== system FaultCheck/FaultDiagnose/IGBTTempDiag/IGBTULowerTempDiag/EnableJudgement ==
  SysSelfCheckDownFlg : Inport
  DiagEn : Inport  Port=2
  Constant : Constant  Value=true
  Logical Operator : Logic  AllPortsSameDT=off  OutDataTypeStr=boolean
  Logical Operator1 : Logic  AllPortsSameDT=off  OutDataTypeStr=boolean
  Logical Operator2 : Logic  AllPortsSameDT=off  OutDataTypeStr=boolean
  DiagEnOut : Outport
  wires:
  Logical Operator1/1 -> Logical Operator2/2
  Constant/1 -> Logical Operator1/1, Logical Operator/1
  DiagEn/1 -> Logical Operator1/2
  SysSelfCheckDownFlg/1 -> Logical Operator/2
  Logical Operator/1 -> Logical Operator2/1
  Logical Operator2/1 -> DiagEnOut/1  "M_Flt_IGBTULowerTempDiagEn_b"

== system FaultCheck/FaultDiagnose/IGBTTempDiag/IGBTULowerTempDiag/FaultLevelDeter ==
  IGBTULowerTempFlgOut : Inport
  FaultLevel : Inport  Port=2
  If : If  IfExpression=u1 == 0
  LowerOne : Subsystem  TreatAsAtomicUnit=on
  Merge : Merge
  Normal : Subsystem  TreatAsAtomicUnit=on
  IGBTULowerTempFltLevelOut : Outport
  wires:
  FaultLevel/1 -> LowerOne/1(FaultLevel)
  Merge/1 -> IGBTULowerTempFltLevelOut/1  "M_Flt_IGBTULowerTempFltLevelOut_u8"
  LowerOne/1(IGBTULowerTempFltLevel) -> Merge/2
  Normal/1(IGBTULowerTempFltLevel) -> Merge/1
  If/2 -> LowerOne/Action
  If/1 -> Normal/Action
  IGBTULowerTempFlgOut/1 -> If/1

== system FaultCheck/FaultDiagnose/IGBTTempDiag/IGBTULowerTempDiag/Parameters ==
  Bus Creator : BusCreator  Inputs=8
  Constant : Constant  Value=C_Flt_IGBTULowerTempTrigTh_s32
  Constant1 : Constant  Value=C_Flt_IGBTULowerTempRecTh_s32
  Constant10 : Constant  Value=C_Flt_IGBTULowerTempRecoveryTh_u16
  Constant11 : Constant  Value=C_Flt_LevelTwo_u8
  Constant2 : Constant  Value=C_Flt_IGBTULowerTempPowerCoeff
  Constant7 : Constant  Value=C_Flt_IGBTULowerTempDiagEn_b
  Constant8 : Constant  Value=C_Flt_IGBTULowerTempErrCode_u16
  Constant9 : Constant  Value=C_Flt_IGBTULowerTempConfirmTh_u16
  Param : Outport
  wires:
  Constant1/1 -> Bus Creator/2  "IGBTULowerTempRecTh"
  Constant2/1 -> Bus Creator/8  "IGBTULowerTempPowerCoeff"
  Constant11/1 -> Bus Creator/7  "IGBTULowerTempFltLevel"
  Constant10/1 -> Bus Creator/6  "IGBTULowerTempRecoveryTh"
  Constant9/1 -> Bus Creator/5  "IGBTULowerTempConfirmTh"
  Constant8/1 -> Bus Creator/4  "IGBTULowerTempErrCode"
  Constant7/1 -> Bus Creator/3  "IGBTULowerTempDiagEn"
  Constant/1 -> Bus Creator/1  "IGBTULowerTempTrigTh"
  Bus Creator/1 -> Param/1

== system FaultCheck/FaultDiagnose/IGBTTempDiag/IGBTULowerTempDiag/PowerReductionCoeffDeter ==
  IGBTULowerTempFltLevelOut : Inport
  PowerCoeff : Inport  Port=2
  If : If  IfExpression=u1 < 2  ElseIfExpressions=u1 == 2
  If Action Subsystem : Subsystem  TreatAsAtomicUnit=on
  If Action Subsystem1 : Subsystem  TreatAsAtomicUnit=on
  If Action Subsystem2 : Subsystem  TreatAsAtomicUnit=on
  Merge : Merge  Inputs=3
  IGBTULowerTempPowerCoeffOut : Outport
  wires:
  Merge/1 -> IGBTULowerTempPowerCoeffOut/1  "M_Flt_IGBTULowerTempPowerCoeffOut_s32"
  If Action Subsystem2/1(Coeff) -> Merge/3
  If Action Subsystem1/1(Coeff) -> Merge/2
  If Action Subsystem/1(Coeff) -> Merge/1
  PowerCoeff/1 -> If Action Subsystem1/1(PowerCoeff)
  If/3 -> If Action Subsystem2/Action
  If/2 -> If Action Subsystem1/Action
  If/1 -> If Action Subsystem/Action
  IGBTULowerTempFltLevelOut/1 -> If/1

== system FaultCheck/FaultDiagnose/IGBTTempDiag/IGBTUOverTempDiag/Diagnose ==
  DiagEnOut : Inport
  IGBTUTemp : Inport  Port=2
  Parameter : Inport  Port=3
  Disable : Subsystem  TreatAsAtomicUnit=on
  If : If  IfExpression=u1 == 0
  Merge : Merge
  NormalDiag : Subsystem  TreatAsAtomicUnit=on
  IGBTUOverTempFlgOut : Outport
  wires:
  DiagEnOut/1 -> If/1
  If/1 -> Disable/Action
  If/2 -> NormalDiag/Action
  IGBTUTemp/1 -> NormalDiag/1(IGBTUTemp)
  Parameter/1 -> NormalDiag/2(Parameter)
  Disable/1(IGBTUOverTempFltDeb) -> Merge/1
  NormalDiag/1(IGBTUOverTempFltDeb) -> Merge/2
  Merge/1 -> IGBTUOverTempFlgOut/1  "M_Flt_IGBTUOverTempFlgOut_b"

== system FaultCheck/FaultDiagnose/IGBTTempDiag/IGBTUOverTempDiag/EnableJudgement ==
  SysSelfCheckDownFlg : Inport
  DiagEn : Inport  Port=2
  Constant : Constant  Value=true
  Logical Operator : Logic  AllPortsSameDT=off  OutDataTypeStr=boolean
  Logical Operator1 : Logic  AllPortsSameDT=off  OutDataTypeStr=boolean
  Logical Operator2 : Logic  AllPortsSameDT=off  OutDataTypeStr=boolean
  DiagEnOut : Outport
  wires:
  Logical Operator2/1 -> DiagEnOut/1  "M_Flt_IGBTUOverTempDiagEn_b"
  Logical Operator/1 -> Logical Operator2/1
  SysSelfCheckDownFlg/1 -> Logical Operator/2
  DiagEn/1 -> Logical Operator1/2
  Constant/1 -> Logical Operator/1, Logical Operator1/1
  Logical Operator1/1 -> Logical Operator2/2

== system FaultCheck/FaultDiagnose/IGBTTempDiag/IGBTUOverTempDiag/FaultLevelDeter ==
  IGBTUOverTempFlgOut : Inport
  FaultLevel : Inport  Port=2
  If : If  IfExpression=u1 == 0
  LowerOne : Subsystem  TreatAsAtomicUnit=on
  Merge : Merge
  Normal : Subsystem  TreatAsAtomicUnit=on
  IGBTUOverTempFltLevelOut : Outport
  wires:
  IGBTUOverTempFlgOut/1 -> If/1
  If/1 -> Normal/Action
  If/2 -> LowerOne/Action
  Normal/1(IGBTUOverTempFltLevel) -> Merge/1
  LowerOne/1(IGBTUOverTempFltLevel) -> Merge/2
  Merge/1 -> IGBTUOverTempFltLevelOut/1  "M_Flt_IGBTUOverTempFltLevelOut_u8"
  FaultLevel/1 -> LowerOne/1(FaultLevel)

== system FaultCheck/FaultDiagnose/IGBTTempDiag/IGBTUOverTempDiag/Parameters ==
  IGBTUTemp : Inport
  1-D Lookup Table1 : Lookup_n-D  NumberOfTableDimensions=1  BreakpointsForDimension1=[-5:5]  BreakpointsForDimension1DataTypeStr=Inherit: Inherit from 'Breakpoint data'  IndexSearchMethod=Linear search  Table=tanh([-5:5])  TableDataTypeStr=Inherit: Inherit from 'Table data'  ExtrapMethod=Clip  UseLastTableValue=on  InternalRulePriority=Speed  OutDataTypeStr=single  RndMeth=Simplest
  Bus Creator : BusCreator  Inputs=8
  Constant : Constant  Value=C_Flt_IGBTUOverTempTrigTh_s32
  Constant1 : Constant  Value=C_Flt_IGBTUOverTempRecTh_s32
  Constant10 : Constant  Value=C_Flt_IGBTUOverTempRecoveryTh_u16
  Constant11 : Constant  Value=C_Flt_LevelTwo_u8
  Constant7 : Constant  Value=C_Flt_IGBTUOverTempDiagEn_b
  Constant8 : Constant  Value=C_Flt_IGBTUOverTempErrCode_u16
  Constant9 : Constant  Value=C_Flt_IGBTUOverTempConfirmTh_u16
  Param : Outport
  wires:
  Bus Creator/1 -> Param/1
  IGBTUTemp/1 -> 1-D Lookup Table1/1
  Constant/1 -> Bus Creator/1  "IGBTUOverTempTrigTh"
  Constant7/1 -> Bus Creator/3  "IGBTUOverTempDiagEn"
  Constant8/1 -> Bus Creator/4  "IGBTUOverTempErrCode"
  Constant9/1 -> Bus Creator/5  "IGBTUOverTempConfirmTh"
  Constant10/1 -> Bus Creator/6  "IGBTUOverTempRecoveryTh"
  Constant11/1 -> Bus Creator/7  "IGBTUOverTempFltLevel"
  1-D Lookup Table1/1 -> Bus Creator/8  "IGBTUOverTempPowerCoeff"
  Constant1/1 -> Bus Creator/2  "IGBTUOverTempRecTh"

== system FaultCheck/FaultDiagnose/IGBTTempDiag/IGBTUOverTempDiag/PowerReductionCoeffDeter ==
  IGBTUOverTempFltLevelOut : Inport
  PowerCoeff : Inport  Port=2
  If : If  IfExpression=u1 < 2  ElseIfExpressions=u1 == 2
  If Action Subsystem : Subsystem  TreatAsAtomicUnit=on
  If Action Subsystem1 : Subsystem  TreatAsAtomicUnit=on
  If Action Subsystem2 : Subsystem  TreatAsAtomicUnit=on
  Merge : Merge  Inputs=3
  IGBTUOverTempPowerCoeffOut : Outport
  wires:
  IGBTUOverTempFltLevelOut/1 -> If/1
  If/1 -> If Action Subsystem/Action
  If/2 -> If Action Subsystem1/Action
  If/3 -> If Action Subsystem2/Action
  PowerCoeff/1 -> If Action Subsystem1/1(PowerCoeff)
  If Action Subsystem/1(Coeff) -> Merge/1
  If Action Subsystem1/1(Coeff) -> Merge/2
  If Action Subsystem2/1(Coeff) -> Merge/3
  Merge/1 -> IGBTUOverTempPowerCoeffOut/1  "M_Flt_IGBTUOverTempPowerCoeffOut_s32"

== system FaultCheck/FaultDiagnose/IGBTTempDiag/IGBTVLowerTempDiag/Diagnose ==
  DiagEnOut : Inport
  IGBTVTemp : Inport  Port=2
  Parameter : Inport  Port=3
  Disable : Subsystem  TreatAsAtomicUnit=on
  If : If  IfExpression=u1 == 0
  Merge : Merge
  NormalDiag : Subsystem  TreatAsAtomicUnit=on
  IGBTVLowerTempFlgOut : Outport
  wires:
  DiagEnOut/1 -> If/1
  If/1 -> Disable/Action
  If/2 -> NormalDiag/Action
  IGBTVTemp/1 -> NormalDiag/1(IGBTVTemp)
  Parameter/1 -> NormalDiag/2(Parameter)
  Disable/1(IGBTVLowerTempFltDeb) -> Merge/1
  NormalDiag/1(IGBTVLowerTempFltDeb) -> Merge/2
  Merge/1 -> IGBTVLowerTempFlgOut/1  "M_Flt_IGBTVLowerTempFlgOut_b"

== system FaultCheck/FaultDiagnose/IGBTTempDiag/IGBTVLowerTempDiag/EnableJudgement ==
  SysSelfCheckDownFlg : Inport
  DiagEn : Inport  Port=2
  Constant : Constant  Value=true
  Logical Operator : Logic  AllPortsSameDT=off  OutDataTypeStr=boolean
  Logical Operator1 : Logic  AllPortsSameDT=off  OutDataTypeStr=boolean
  Logical Operator2 : Logic  AllPortsSameDT=off  OutDataTypeStr=boolean
  DiagEnOut : Outport
  wires:
  Logical Operator2/1 -> DiagEnOut/1  "M_Flt_IGBTVLowerTempDiagEn_b"
  Logical Operator/1 -> Logical Operator2/1
  SysSelfCheckDownFlg/1 -> Logical Operator/2
  DiagEn/1 -> Logical Operator1/2
  Constant/1 -> Logical Operator/1, Logical Operator1/1
  Logical Operator1/1 -> Logical Operator2/2

== system FaultCheck/FaultDiagnose/IGBTTempDiag/IGBTVLowerTempDiag/FaultLevelDeter ==
  IGBTVLowerTempFlgOut : Inport
  FaultLevel : Inport  Port=2
  If : If  IfExpression=u1 == 0
  LowerOne : Subsystem  TreatAsAtomicUnit=on
  Merge : Merge
  Normal : Subsystem  TreatAsAtomicUnit=on
  IGBTVLowerTempFltLevelOut : Outport
  wires:
  IGBTVLowerTempFlgOut/1 -> If/1
  If/1 -> Normal/Action
  If/2 -> LowerOne/Action
  Normal/1(IGBTVLowerTempFltLevel) -> Merge/1
  LowerOne/1(IGBTVLowerTempFltLevel) -> Merge/2
  Merge/1 -> IGBTVLowerTempFltLevelOut/1  "M_Flt_IGBTVLowerTempFltLevelOut_u8"
  FaultLevel/1 -> LowerOne/1(FaultLevel)

== system FaultCheck/FaultDiagnose/IGBTTempDiag/IGBTVLowerTempDiag/Parameters ==
  Bus Creator : BusCreator  Inputs=8
  Constant : Constant  Value=C_Flt_IGBTVLowerTempTrigTh_s32
  Constant1 : Constant  Value=C_Flt_IGBTVLowerTempRecTh_s32
  Constant10 : Constant  Value=C_Flt_IGBTVLowerTempRecoveryTh_u16
  Constant11 : Constant  Value=C_Flt_LevelTwo_u8
  Constant2 : Constant  Value=C_Flt_IGBTVLowerTempPowerCoeff
  Constant7 : Constant  Value=C_Flt_IGBTVLowerTempDiagEn_b
  Constant8 : Constant  Value=C_Flt_IGBTVLowerTempErrCode_u16
  Constant9 : Constant  Value=C_Flt_IGBTVLowerTempConfirmTh_u16
  Param : Outport
  wires:
  Bus Creator/1 -> Param/1
  Constant/1 -> Bus Creator/1  "IGBTVLowerTempTrigTh"
  Constant7/1 -> Bus Creator/3  "IGBTVLowerTempDiagEn"
  Constant8/1 -> Bus Creator/4  "IGBTVLowerTempErrCode"
  Constant9/1 -> Bus Creator/5  "IGBTVLowerTempConfirmTh"
  Constant10/1 -> Bus Creator/6  "IGBTVLowerTempRecoveryTh"
  Constant11/1 -> Bus Creator/7  "IGBTVLowerTempFltLevel"
  Constant2/1 -> Bus Creator/8  "IGBTVLowerTempPowerCoeff"
  Constant1/1 -> Bus Creator/2  "IGBTVLowerTempRecTh"

== system FaultCheck/FaultDiagnose/IGBTTempDiag/IGBTVLowerTempDiag/PowerReductionCoeffDeter ==
  IGBTVLowerTempFltLevelOut : Inport
  PowerCoeff : Inport  Port=2
  If : If  IfExpression=u1 < 2  ElseIfExpressions=u1 == 2
  If Action Subsystem : Subsystem  TreatAsAtomicUnit=on
  If Action Subsystem1 : Subsystem  TreatAsAtomicUnit=on
  If Action Subsystem2 : Subsystem  TreatAsAtomicUnit=on
  Merge : Merge  Inputs=3
  IGBTVLowerTempPowerCoeffOut : Outport
  wires:
  IGBTVLowerTempFltLevelOut/1 -> If/1
  If/1 -> If Action Subsystem/Action
  If/2 -> If Action Subsystem1/Action
  If/3 -> If Action Subsystem2/Action
  PowerCoeff/1 -> If Action Subsystem1/1(PowerCoeff)
  If Action Subsystem/1(Coeff) -> Merge/1
  If Action Subsystem1/1(Coeff) -> Merge/2
  If Action Subsystem2/1(Coeff) -> Merge/3
  Merge/1 -> IGBTVLowerTempPowerCoeffOut/1  "M_Flt_IGBTVLowerTempPowerCoeffOut_s32"

== system FaultCheck/FaultDiagnose/IGBTTempDiag/IGBTVOverTempDiag/Diagnose ==
  DiagEnOut : Inport
  IGBTVTemp : Inport  Port=2
  Parameter : Inport  Port=3
  Disable : Subsystem  TreatAsAtomicUnit=on
  If : If  IfExpression=u1 == 0
  Merge : Merge
  NormalDiag : Subsystem  TreatAsAtomicUnit=on
  IGBTVOverTempFlgOut : Outport
  wires:
  Merge/1 -> IGBTVOverTempFlgOut/1  "M_Flt_IGBTVOverTempFlgOut_b"
  NormalDiag/1(IGBTVOverTempFltDeb) -> Merge/2
  Disable/1(IGBTVOverTempFltDeb) -> Merge/1
  Parameter/1 -> NormalDiag/2(Parameter)
  IGBTVTemp/1 -> NormalDiag/1(IGBTVTemp)
  If/2 -> NormalDiag/Action
  If/1 -> Disable/Action
  DiagEnOut/1 -> If/1

== system FaultCheck/FaultDiagnose/IGBTTempDiag/IGBTVOverTempDiag/EnableJudgement ==
  SysSelfCheckDownFlg : Inport
  DiagEn : Inport  Port=2
  Constant : Constant  Value=true
  Logical Operator : Logic  AllPortsSameDT=off  OutDataTypeStr=boolean
  Logical Operator1 : Logic  AllPortsSameDT=off  OutDataTypeStr=boolean
  Logical Operator2 : Logic  AllPortsSameDT=off  OutDataTypeStr=boolean
  DiagEnOut : Outport
  wires:
  Logical Operator1/1 -> Logical Operator2/2
  Constant/1 -> Logical Operator1/1, Logical Operator/1
  DiagEn/1 -> Logical Operator1/2
  SysSelfCheckDownFlg/1 -> Logical Operator/2
  Logical Operator/1 -> Logical Operator2/1
  Logical Operator2/1 -> DiagEnOut/1  "M_Flt_IGBTVOverTempDiagEn_b"

== system FaultCheck/FaultDiagnose/IGBTTempDiag/IGBTVOverTempDiag/FaultLevelDeter ==
  IGBTVOverTempFlgOut : Inport
  FaultLevel : Inport  Port=2
  If : If  IfExpression=u1 == 0
  LowerOne : Subsystem  TreatAsAtomicUnit=on
  Merge : Merge
  Normal : Subsystem  TreatAsAtomicUnit=on
  IGBTVOverTempFltLevelOut : Outport
  wires:
  FaultLevel/1 -> LowerOne/1(FaultLevel)
  Merge/1 -> IGBTVOverTempFltLevelOut/1  "M_Flt_IGBTVOverTempFltLevelOut_u8"
  LowerOne/1(IGBTVOverTempFltLevel) -> Merge/2
  Normal/1(IGBTVOverTempFltLevel) -> Merge/1
  If/2 -> LowerOne/Action
  If/1 -> Normal/Action
  IGBTVOverTempFlgOut/1 -> If/1

== system FaultCheck/FaultDiagnose/IGBTTempDiag/IGBTVOverTempDiag/Parameters ==
  IGBTVTemp : Inport
  1-D Lookup Table1 : Lookup_n-D  NumberOfTableDimensions=1  BreakpointsForDimension1=[-5:5]  BreakpointsForDimension1DataTypeStr=Inherit: Inherit from 'Breakpoint data'  IndexSearchMethod=Linear search  Table=tanh([-5:5])  TableDataTypeStr=Inherit: Inherit from 'Table data'  ExtrapMethod=Clip  UseLastTableValue=on  InternalRulePriority=Speed  OutDataTypeStr=single  RndMeth=Simplest
  Bus Creator : BusCreator  Inputs=8
  Constant : Constant  Value=C_Flt_IGBTVOverTempTrigTh_s32
  Constant1 : Constant  Value=C_Flt_IGBTVOverTempRecTh_s32
  Constant10 : Constant  Value=C_Flt_IGBTVOverTempRecoveryTh_u16
  Constant11 : Constant  Value=C_Flt_LevelTwo_u8
  Constant7 : Constant  Value=C_Flt_IGBTVOverTempDiagEn_b
  Constant8 : Constant  Value=C_Flt_IGBTVOverTempErrCode_u16
  Constant9 : Constant  Value=C_Flt_IGBTVOverTempConfirmTh_u16
  Param : Outport
  wires:
  Constant1/1 -> Bus Creator/2  "IGBTVOverTempRecTh"
  1-D Lookup Table1/1 -> Bus Creator/8  "IGBTVOverTempPowerCoeff"
  Constant11/1 -> Bus Creator/7  "IGBTVOverTempFltLevel"
  Constant10/1 -> Bus Creator/6  "IGBTVOverTempRecoveryTh"
  Constant9/1 -> Bus Creator/5  "IGBTVOverTempConfirmTh"
  Constant8/1 -> Bus Creator/4  "IGBTVOverTempErrCode"
  Constant7/1 -> Bus Creator/3  "IGBTVOverTempDiagEn"
  Constant/1 -> Bus Creator/1  "IGBTVOverTempTrigTh"
  IGBTVTemp/1 -> 1-D Lookup Table1/1
  Bus Creator/1 -> Param/1

== system FaultCheck/FaultDiagnose/IGBTTempDiag/IGBTVOverTempDiag/PowerReductionCoeffDeter ==
  IGBTVOverTempFltLevelOut : Inport
  PowerCoeff : Inport  Port=2
  If : If  IfExpression=u1 < 2  ElseIfExpressions=u1 == 2
  If Action Subsystem : Subsystem  TreatAsAtomicUnit=on
  If Action Subsystem1 : Subsystem  TreatAsAtomicUnit=on
  If Action Subsystem2 : Subsystem  TreatAsAtomicUnit=on
  Merge : Merge  Inputs=3
  IGBTVOverTempPowerCoeffOut : Outport
  wires:
  Merge/1 -> IGBTVOverTempPowerCoeffOut/1  "M_Flt_IGBTVOverTempPowerCoeffOut_s32"
  If Action Subsystem2/1(Coeff) -> Merge/3
  If Action Subsystem1/1(Coeff) -> Merge/2
  If Action Subsystem/1(Coeff) -> Merge/1
  PowerCoeff/1 -> If Action Subsystem1/1(PowerCoeff)
  If/3 -> If Action Subsystem2/Action
  If/2 -> If Action Subsystem1/Action
  If/1 -> If Action Subsystem/Action
  IGBTVOverTempFltLevelOut/1 -> If/1

== system FaultCheck/FaultDiagnose/IGBTTempDiag/IGBTWLowerTempDiag/Diagnose ==
  DiagEnOut : Inport
  IGBTWTemp : Inport  Port=2
  Parameter : Inport  Port=3
  Disable : Subsystem  TreatAsAtomicUnit=on
  If : If  IfExpression=u1 == 0
  Merge : Merge
  NormalDiag : Subsystem  TreatAsAtomicUnit=on
  IGBTWLowerTempFlgOut : Outport
  wires:
  DiagEnOut/1 -> If/1
  If/1 -> Disable/Action
  If/2 -> NormalDiag/Action
  IGBTWTemp/1 -> NormalDiag/1(IGBTWTemp)
  Parameter/1 -> NormalDiag/2(Parameter)
  Disable/1(IGBTWLowerTempFltDeb) -> Merge/1
  NormalDiag/1(IGBTWLowerTempFltDeb) -> Merge/2
  Merge/1 -> IGBTWLowerTempFlgOut/1  "M_Flt_IGBTWLowerTempFlgOut_b"

== system FaultCheck/FaultDiagnose/IGBTTempDiag/IGBTWLowerTempDiag/EnableJudgement ==
  SysSelfCheckDownFlg : Inport
  DiagEn : Inport  Port=2
  Constant : Constant  Value=true
  Logical Operator : Logic  AllPortsSameDT=off  OutDataTypeStr=boolean
  Logical Operator1 : Logic  AllPortsSameDT=off  OutDataTypeStr=boolean
  Logical Operator2 : Logic  AllPortsSameDT=off  OutDataTypeStr=boolean
  DiagEnOut : Outport
  wires:
  Logical Operator2/1 -> DiagEnOut/1  "M_Flt_IGBTWLowerTempDiagEn_b"
  Logical Operator/1 -> Logical Operator2/1
  SysSelfCheckDownFlg/1 -> Logical Operator/2
  DiagEn/1 -> Logical Operator1/2
  Constant/1 -> Logical Operator/1, Logical Operator1/1
  Logical Operator1/1 -> Logical Operator2/2

== system FaultCheck/FaultDiagnose/IGBTTempDiag/IGBTWLowerTempDiag/FaultLevelDeter ==
  IGBTWLowerTempFlgOut : Inport
  FaultLevel : Inport  Port=2
  If : If  IfExpression=u1 == 0
  LowerOne : Subsystem  TreatAsAtomicUnit=on
  Merge : Merge
  Normal : Subsystem  TreatAsAtomicUnit=on
  IGBTWLowerTempFltLevelOut : Outport
  wires:
  IGBTWLowerTempFlgOut/1 -> If/1
  If/1 -> Normal/Action
  If/2 -> LowerOne/Action
  Normal/1(IGBTWLowerTempFltLevel) -> Merge/1
  LowerOne/1(IGBTWLowerTempFltLevel) -> Merge/2
  Merge/1 -> IGBTWLowerTempFltLevelOut/1  "M_Flt_IGBTWLowerTempFltLevelOut_u8"
  FaultLevel/1 -> LowerOne/1(FaultLevel)

== system FaultCheck/FaultDiagnose/IGBTTempDiag/IGBTWLowerTempDiag/Parameters ==
  Bus Creator : BusCreator  Inputs=8
  Constant : Constant  Value=C_Flt_IGBTWLowerTempTrigTh_s32
  Constant1 : Constant  Value=C_Flt_IGBTWLowerTempRecTh_s32
  Constant10 : Constant  Value=C_Flt_IGBTWLowerTempRecoveryTh_u16
  Constant11 : Constant  Value=C_Flt_LevelTwo_u8
  Constant2 : Constant  Value=C_Flt_IGBTWLowerTempPowerCoeff
  Constant7 : Constant  Value=C_Flt_IGBTWLowerTempDiagEn_b
  Constant8 : Constant  Value=C_Flt_IGBTWLowerTempErrCode_u16
  Constant9 : Constant  Value=C_Flt_IGBTWLowerTempConfirmTh_u16
  Param : Outport
  wires:
  Bus Creator/1 -> Param/1
  Constant/1 -> Bus Creator/1  "IGBTWLowerTempTrigTh"
  Constant7/1 -> Bus Creator/3  "IGBTWLowerTempDiagEn"
  Constant8/1 -> Bus Creator/4  "IGBTWLowerTempErrCode"
  Constant9/1 -> Bus Creator/5  "IGBTWLowerTempConfirmTh"
  Constant10/1 -> Bus Creator/6  "IGBTWLowerTempRecoveryTh"
  Constant11/1 -> Bus Creator/7  "IGBTWLowerTempFltLevel"
  Constant2/1 -> Bus Creator/8  "IGBTWLowerTempPowerCoeff"
  Constant1/1 -> Bus Creator/2  "IGBTWLowerTempRecTh"

== system FaultCheck/FaultDiagnose/IGBTTempDiag/IGBTWLowerTempDiag/PowerReductionCoeffDeter ==
  IGBTWLowerTempFltLevelOut : Inport
  PowerCoeff : Inport  Port=2
  If : If  IfExpression=u1 < 2  ElseIfExpressions=u1 == 2
  If Action Subsystem : Subsystem  TreatAsAtomicUnit=on
  If Action Subsystem1 : Subsystem  TreatAsAtomicUnit=on
  If Action Subsystem2 : Subsystem  TreatAsAtomicUnit=on
  Merge : Merge  Inputs=3
  IGBTWLowerTempPowerCoeffOut : Outport
  wires:
  IGBTWLowerTempFltLevelOut/1 -> If/1
  If/1 -> If Action Subsystem/Action
  If/2 -> If Action Subsystem1/Action
  If/3 -> If Action Subsystem2/Action
  PowerCoeff/1 -> If Action Subsystem1/1(PowerCoeff)
  If Action Subsystem/1(Coeff) -> Merge/1
  If Action Subsystem1/1(Coeff) -> Merge/2
  If Action Subsystem2/1(Coeff) -> Merge/3
  Merge/1 -> IGBTWLowerTempPowerCoeffOut/1  "M_Flt_IGBTWLowerTempPowerCoeffOut_s32"

== system FaultCheck/FaultDiagnose/IGBTTempDiag/IGBTWOverTempDiag/Diagnose ==
  DiagEnOut : Inport
  IGBTWTemp : Inport  Port=2
  Parameter : Inport  Port=3
  Disable : Subsystem  TreatAsAtomicUnit=on
  If : If  IfExpression=u1 == 0
  Merge : Merge
  NormalDiag : Subsystem  TreatAsAtomicUnit=on
  IGBTWOverTempFlgOut : Outport
  wires:
  DiagEnOut/1 -> If/1
  If/1 -> Disable/Action
  If/2 -> NormalDiag/Action
  IGBTWTemp/1 -> NormalDiag/1(IGBTWTemp)
  Parameter/1 -> NormalDiag/2(Parameter)
  Disable/1(IGBTWOverTempFltDeb) -> Merge/1
  NormalDiag/1(IGBTWOverTempFltDeb) -> Merge/2
  Merge/1 -> IGBTWOverTempFlgOut/1  "M_Flt_IGBTWOverTempFlgOut_b"

== system FaultCheck/FaultDiagnose/IGBTTempDiag/IGBTWOverTempDiag/EnableJudgement ==
  SysSelfCheckDownFlg : Inport
  DiagEn : Inport  Port=2
  Constant : Constant  Value=true
  Logical Operator : Logic  AllPortsSameDT=off  OutDataTypeStr=boolean
  Logical Operator1 : Logic  AllPortsSameDT=off  OutDataTypeStr=boolean
  Logical Operator2 : Logic  AllPortsSameDT=off  OutDataTypeStr=boolean
  DiagEnOut : Outport
  wires:
  Logical Operator2/1 -> DiagEnOut/1  "M_Flt_IGBTWOverTempDiagEn_b"
  Logical Operator/1 -> Logical Operator2/1
  SysSelfCheckDownFlg/1 -> Logical Operator/2
  DiagEn/1 -> Logical Operator1/2
  Constant/1 -> Logical Operator/1, Logical Operator1/1
  Logical Operator1/1 -> Logical Operator2/2

== system FaultCheck/FaultDiagnose/IGBTTempDiag/IGBTWOverTempDiag/FaultLevelDeter ==
  IGBTWOverTempFlgOut : Inport
  FaultLevel : Inport  Port=2
  If : If  IfExpression=u1 == 0
  LowerOne : Subsystem  TreatAsAtomicUnit=on
  Merge : Merge
  Normal : Subsystem  TreatAsAtomicUnit=on
  IGBTWOverTempFltLevelOut : Outport
  wires:
  IGBTWOverTempFlgOut/1 -> If/1
  If/1 -> Normal/Action
  If/2 -> LowerOne/Action
  Normal/1(IGBTWOverTempFltLevel) -> Merge/1
  LowerOne/1(IGBTWOverTempFltLevel) -> Merge/2
  Merge/1 -> IGBTWOverTempFltLevelOut/1  "M_Flt_IGBTWOverTempFltLevelOut_u8"
  FaultLevel/1 -> LowerOne/1(FaultLevel)

== system FaultCheck/FaultDiagnose/IGBTTempDiag/IGBTWOverTempDiag/Parameters ==
  IGBTWTemp : Inport
  1-D Lookup Table1 : Lookup_n-D  NumberOfTableDimensions=1  BreakpointsForDimension1=[-5:5]  BreakpointsForDimension1DataTypeStr=Inherit: Inherit from 'Breakpoint data'  IndexSearchMethod=Linear search  Table=tanh([-5:5])  TableDataTypeStr=Inherit: Inherit from 'Table data'  ExtrapMethod=Clip  UseLastTableValue=on  InternalRulePriority=Speed  OutDataTypeStr=single  RndMeth=Simplest
  Bus Creator : BusCreator  Inputs=8
  Constant : Constant  Value=C_Flt_IGBTWOverTempTrigTh_s32
  Constant1 : Constant  Value=C_Flt_IGBTWOverTempRecTh_s32
  Constant10 : Constant  Value=C_Flt_IGBTWOverTempRecoveryTh_u16
  Constant11 : Constant  Value=C_Flt_LevelTwo_u8
  Constant7 : Constant  Value=C_Flt_IGBTWOverTempDiagEn_b
  Constant8 : Constant  Value=C_Flt_IGBTWOverTempErrCode_u16
  Constant9 : Constant  Value=C_Flt_IGBTWOverTempConfirmTh_u16
  Param : Outport
  wires:
  Bus Creator/1 -> Param/1
  IGBTWTemp/1 -> 1-D Lookup Table1/1
  Constant/1 -> Bus Creator/1  "IGBTWOverTempTrigTh"
  Constant7/1 -> Bus Creator/3  "IGBTWOverTempDiagEn"
  Constant8/1 -> Bus Creator/4  "IGBTWOverTempErrCode"
  Constant9/1 -> Bus Creator/5  "IGBTWOverTempConfirmTh"
  Constant10/1 -> Bus Creator/6  "IGBTWOverTempRecoveryTh"
  Constant11/1 -> Bus Creator/7  "IGBTWOverTempFltLevel"
  1-D Lookup Table1/1 -> Bus Creator/8  "IGBTWOverTempPowerCoeff"
  Constant1/1 -> Bus Creator/2  "IGBTWOverTempRecTh"
